simulink model "model"  (R2016b)
settings: Solver=VariableStepAuto  StartTime=0.0  StopTime=par.t12  FixedStep=0.001  RelTol=1e-6
StartFcn:
  | tic;
StopFcn:
  | toc;
values from neighbouring files (symbols this model uses):
  as = rmfield(as,'data')    [PrepareForModel (2).m]    (also in PrepareForModel.m)
  trj = rmfield(trj,'aerodata')    [ImportFromMatAndExcel.m]
undefined symbols (not defined in the file or in its folder): dm
libraries: aerolibschedule x5, simulink_extras x2
settings Model: Creator=admin  LastModifiedBy=ivan_
settings SolverCC: PositivePriorityOrder=on  AutoInsertRateTranBlk=on
settings DataIOCC: LimitDataPoints=on  SaveFormat=Array
settings OptimizationCC: LifeSpan=inf
settings DebuggingCC: SFUnexpectedBacktrackingDiag=warning  SFNoUnconditionalDefaultTransitionDiag=warning  SFExecutionAtInitializationDiag=none
settings HardwareCC: ProdBitPerPointer=32  ProdBitPerSizeT=32  ProdBitPerPtrDiffT=32  ProdLargestAtomicFloat=None  ProdIntDivRoundTo=Undefined  ProdEndianess=Unspecified  ProdWordSize=32  ProdHWDeviceType=32-bit Generic
settings ModelReferenceCC: PropagateSignalLabelsOutOfModel=off
settings GRTTargetCC: TargetLangStandard=C89/C90 (ANSI)  GeneratePreprocessorConditionals=Disable all
settings ConfigComp: CovMetricSettings=dw  CovHtmlReporting=on  CovSaveCumulativeToWorkspaceVar=on  CovSaveSingleToWorkspaceVar=on  CovExternalEMLEnable=off  CovSFcnEnable=off

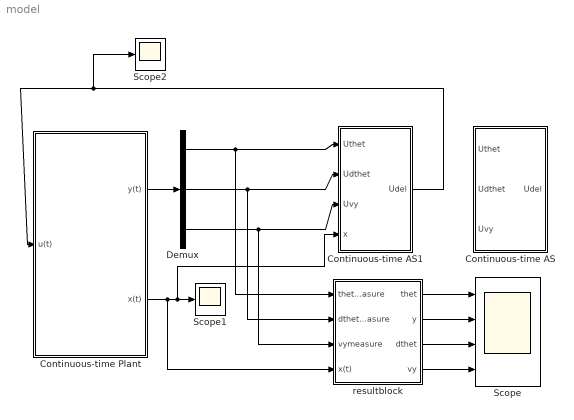
== system model ==
  Continuous-time Plant : Subsystem  VariantControl=Variant
  Continuous-time AS : Subsystem  VariantControl=Variant1
  Continuous-time AS1 : Subsystem  VariantControl=Variant1
  Demux : Demux  Outputs=3
  Scope : Scope  NumInputPorts=4
  Scope1 : Scope
  Scope2 : Scope
  resultblock : Subsystem
  wires:
  Demux/1 -> Continuous-time AS1/1(Uthet), resultblock/1(thetmeasure)
  Demux/2 -> Continuous-time AS1/2(Udthet), resultblock/2(dthetmeasure)
  Demux/3 -> Continuous-time AS1/3(Uvy), resultblock/3(vymeasure)
  Continuous-time Plant/1(y(t)) -> Demux/1
  resultblock/1(thet) -> Scope/1
  resultblock/2(y) -> Scope/2
  resultblock/3(dthet) -> Scope/3
  resultblock/4(vy) -> Scope/4
  Continuous-time Plant/2(x(t)) -> Continuous-time AS1/4("x "), Scope1/1, resultblock/4(x(t))
  Continuous-time AS1/1(Udel) -> Scope2/1, Continuous-time Plant/1(u(t))

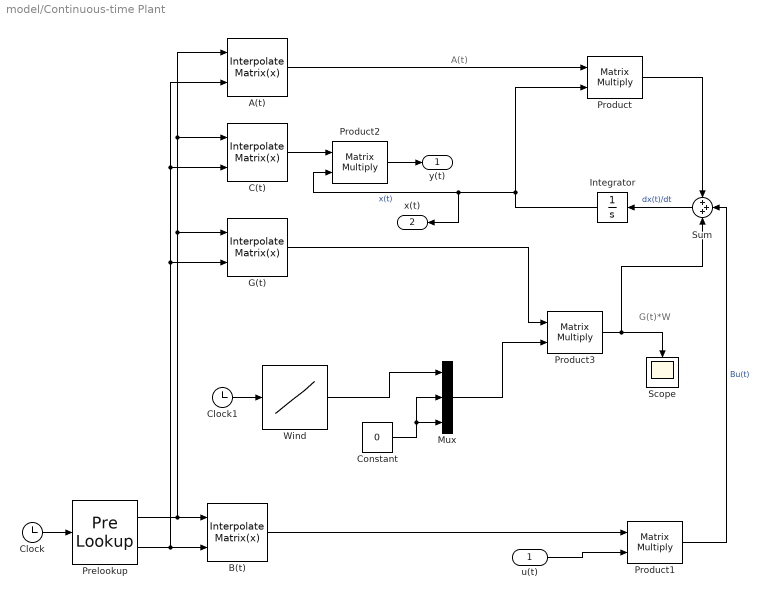
== system model/Continuous-time Plant ==
  note: G(t)*W
  note: A(t)
  u(t) : Inport
  "A(t) " : aerolibschedule/Interpolate Matrix(x)   matrix=dm.A
  B(t) : aerolibschedule/Interpolate Matrix(x)   matrix=dm.B
  C(t) : aerolibschedule/Interpolate Matrix(x)   matrix=dm.C
  Clock : Clock
  Clock1 : Clock
  Constant : Constant  Value=0
  G(t) : aerolibschedule/Interpolate Matrix(x)   matrix=dm.G
  Integrator : Integrator
  Mux : Mux  Inputs=3
  Prelookup : PreLookup  BreakpointsData=dm.t
  Product{,1..3} (4 alike) : Product  Multiplication=Matrix(*)
  Scope : Scope
  Sum : Sum  Inputs=+++
  Wind : Lookup_n-D  NumberOfTableDimensions=1  BreakpointsForDimension1=dm.t  Table=trj.wind  ExtrapMethod=Clip  UseLastTableValue=on  InternalRulePriority=Speed  RndMeth=Simplest  InputSameDT=on
  y(t) : Outport
  x(t) : Outport  Port=2
  wires:
  Sum/1 -> Integrator/1  "dx(t)/dt"
  u(t)/1 -> Product1/2
  Integrator/1 -> Product2/2, x(t)/1, Product/2  "x(t)"
  Product2/1 -> y(t)/1
  Mux/1 -> Product3/2
  Product3/1 -> Sum/3, Scope/1
  G(t)/1 -> Product3/1
  "A(t) "/1 -> Product/1
  B(t)/1 -> Product1/1
  C(t)/1 -> Product2/1
  Wind/1 -> Mux/1
  Prelookup/2 -> "A(t) "/2, C(t)/2, G(t)/2, B(t)/2
  Prelookup/1 -> "A(t) "/1, C(t)/1, G(t)/1, B(t)/1
  Clock/1 -> Prelookup/1
  Product/1 -> Sum/1
  Clock1/1 -> Wind/1
  Product1/1 -> Sum/2  "Bu(t)"
  Constant/1 -> Mux/3, Mux/2

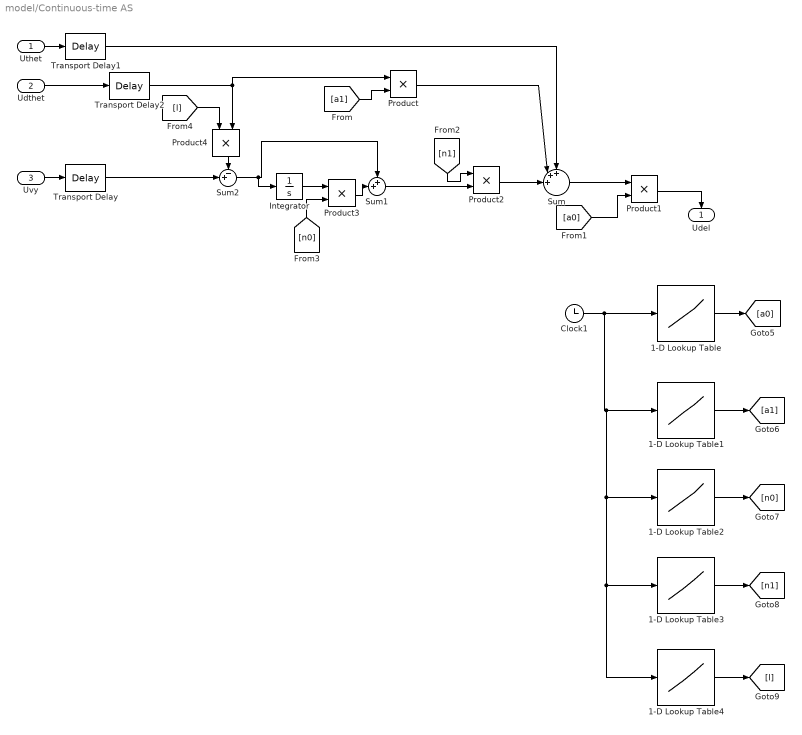
== system model/Continuous-time AS ==
  Uthet : Inport
  Udthet : Inport  Port=2
  Uvy : Inport  Port=3
  1-D Lookup Table : Lookup_n-D  NumberOfTableDimensions=1  BreakpointsForDimension1=as.t  Table=as.a0  ExtrapMethod=Clip  UseLastTableValue=on  InternalRulePriority=Speed  RndMeth=Simplest  InputSameDT=on
  1-D Lookup Table1 : Lookup_n-D  NumberOfTableDimensions=1  BreakpointsForDimension1=as.t  Table=as.a1  ExtrapMethod=Clip  UseLastTableValue=on  InternalRulePriority=Speed  RndMeth=Simplest  InputSameDT=on
  1-D Lookup Table2 : Lookup_n-D  NumberOfTableDimensions=1  BreakpointsForDimension1=as.t  Table=as.n0  ExtrapMethod=Clip  UseLastTableValue=on  InternalRulePriority=Speed  RndMeth=Simplest  InputSameDT=on
  1-D Lookup Table3 : Lookup_n-D  NumberOfTableDimensions=1  BreakpointsForDimension1=as.t  Table=as.n1  ExtrapMethod=Clip  UseLastTableValue=on  InternalRulePriority=Speed  RndMeth=Simplest  InputSameDT=on
  1-D Lookup Table4 : Lookup_n-D  NumberOfTableDimensions=1  BreakpointsForDimension1=as.t  Table=as.l  ExtrapMethod=Clip  UseLastTableValue=on  InternalRulePriority=Speed  RndMeth=Simplest  InputSameDT=on
  Clock1 : Clock
  Integrator : Integrator
  Product{,1..4} (5 alike) : Product
  Sum : Sum  Inputs=+++||
  Sum1 : Sum  Inputs=++|
  Sum2 : Sum  Inputs=-+|
  Transport Delay : TransportDelay  DelayTime=[0.0214]
  Transport Delay1 : TransportDelay  DelayTime=[0.0214]
  Transport Delay2 : TransportDelay  DelayTime=[0.0114]
  Udel : Outport
  wires:
  Sum2/1 -> Integrator/1, Sum1/1
  Sum1/1 -> Product2/2
  Udthet/1 -> Transport Delay2/1
  Sum/1 -> Product1/1
  Product4/1 -> Sum2/1
  Product/1 -> Sum/2
  Uvy/1 -> Transport Delay/1
  Uthet/1 -> Transport Delay1/1
  [a1] -> Product/2
  [a0] -> Product1/2
  Product2/1 -> Sum/3
  Product1/1 -> Udel/1
  [l] -> Product4/1
  [n1] -> Product2/1
  1-D Lookup Table/1 -> [a0]
  1-D Lookup Table1/1 -> [a1]
  1-D Lookup Table2/1 -> [n0]
  1-D Lookup Table3/1 -> [n1]
  1-D Lookup Table4/1 -> [l]
  Clock1/1 -> 1-D Lookup Table4/1, 1-D Lookup Table3/1, 1-D Lookup Table2/1, 1-D Lookup Table1/1, 1-D Lookup Table/1
  [n0] -> Product3/2
  Integrator/1 -> Product3/1
  Product3/1 -> Sum1/2
  Transport Delay/1 -> Sum2/2
  Transport Delay1/1 -> Sum/1
  Transport Delay2/1 -> Product4/2, Product/1

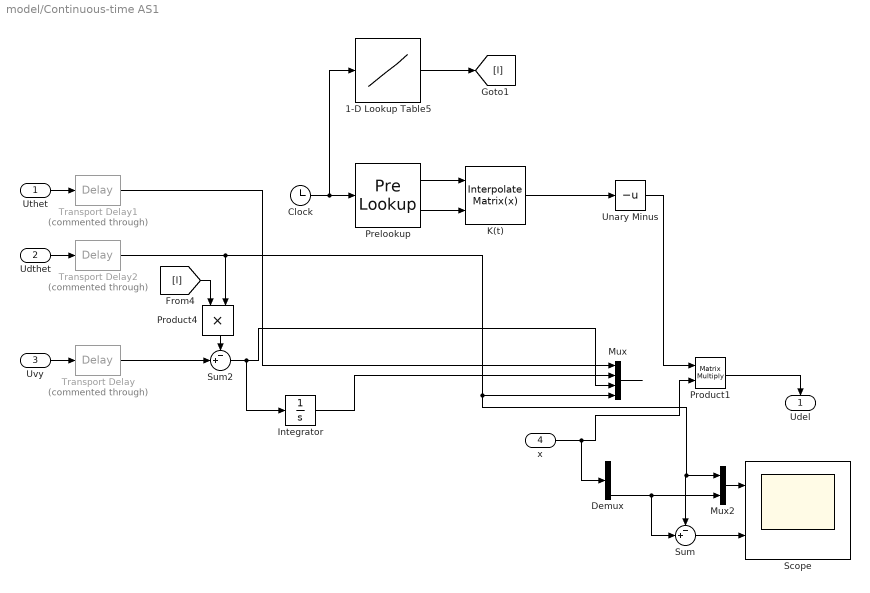
== system model/Continuous-time AS1 ==
  Uthet : Inport
  Udthet : Inport  Port=2
  Uvy : Inport  Port=3
  "x " : Inport  Port=4
  1-D Lookup Table5 : Lookup_n-D  NumberOfTableDimensions=1  BreakpointsForDimension1=as.t  Table=as.l  ExtrapMethod=Clip  UseLastTableValue=on  InternalRulePriority=Speed  RndMeth=Simplest  InputSameDT=on
  Clock : Clock
  Demux : Demux
  Integrator : Integrator
  K(t) : aerolibschedule/Interpolate Matrix(x)   matrix=as.k
  Mux : Mux
  Mux2 : Mux  Inputs=2
  Prelookup : PreLookup  BreakpointsData=dm.t
  Product1 : Product  Multiplication=Matrix(*)
  Product4 : Product
  Scope : Scope  NumInputPorts=2
  Sum : Sum  Inputs=-+|
  Sum2 : Sum  Inputs=-+|
  Transport Delay : TransportDelay  Commented=through  DelayTime=[0.0214]
  Transport Delay1 : TransportDelay  Commented=through  DelayTime=[0.0214]
  Transport Delay2 : TransportDelay  Commented=through  DelayTime=[0.0114]
  Unary Minus : UnaryMinus
  Udel : Outport
  wires:
  Udthet/1 -> Transport Delay2/1
  Product4/1 -> Sum2/1
  Uvy/1 -> Transport Delay/1
  Uthet/1 -> Transport Delay1/1
  K(t)/1 -> Unary Minus/1
  Product1/1 -> Udel/1
  [l] -> Product4/1
  Transport Delay/1 -> Sum2/2
  Transport Delay2/1 -> Product4/2, Sum/1, Mux2/1, Mux/4
  Prelookup/2 -> K(t)/2
  Prelookup/1 -> K(t)/1
  Clock/1 -> 1-D Lookup Table5/1, Prelookup/1
  1-D Lookup Table5/1 -> [l]
  Transport Delay1/1 -> Mux/1
  Integrator/1 -> Mux/2
  Mux/1 -> ?
  Unary Minus/1 -> Product1/1
  "x "/1 -> Demux/1, Product1/2
  Sum2/1 -> Integrator/1, Mux/3
  Demux/4 -> Mux2/2, Sum/2
  Mux2/1 -> Scope/1
  Sum/1 -> Scope/2

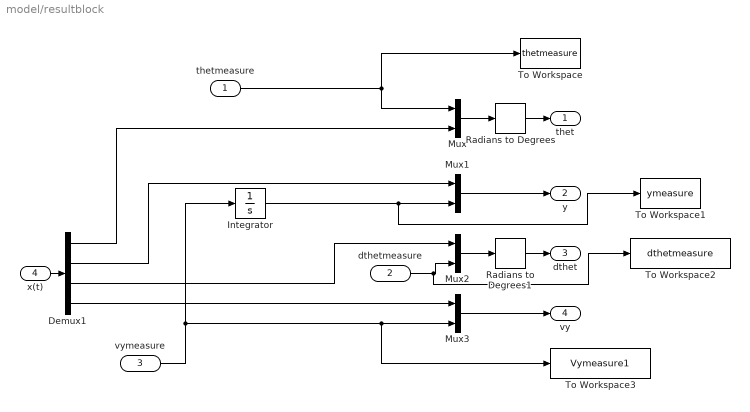
== system model/resultblock ==
  thetmeasure : Inport
  dthetmeasure : Inport  Port=2
  vymeasure : Inport  Port=3
  x(t) : Inport  Port=4
  Demux1 : Demux
  Integrator : Integrator
  Mux{,1..3} (4 alike) : Mux  Inputs=2
  Radians to Degrees : simulink_extras/Transformations/Radians to Degrees
  Radians to Degrees1 : simulink_extras/Transformations/Radians to Degrees
  To Workspace : ToWorkspace  VariableName=thetmeasure  SaveFormat=Structure With Time  SampleTime=-1
  To Workspace1 : ToWorkspace  VariableName=ymeasure  SaveFormat=Structure With Time  SampleTime=-1
  To Workspace2 : ToWorkspace  VariableName=dthetmeasure  SaveFormat=Structure With Time  SampleTime=-1
  To Workspace3 : ToWorkspace  VariableName=Vymeasure1  SaveFormat=Structure With Time  SampleTime=-1
  thet : Outport
  y : Outport  Port=2
  dthet : Outport  Port=3
  vy : Outport  Port=4
  wires:
  x(t)/1 -> Demux1/1
  thetmeasure/1 -> Mux/1, To Workspace/1
  Integrator/1 -> To Workspace1/1, Mux1/2
  dthetmeasure/1 -> To Workspace2/1, Mux2/2
  Demux1/2 -> Mux1/1
  Demux1/3 -> Mux2/1
  Mux/1 -> Radians to Degrees/1
  Demux1/1 -> Mux/2
  Mux3/1 -> vy/1
  Demux1/4 -> Mux3/1
  vymeasure/1 -> Integrator/1, To Workspace3/1, Mux3/2
  Mux1/1 -> y/1
  Mux2/1 -> Radians to Degrees1/1
  Radians to Degrees1/1 -> dthet/1
  Radians to Degrees/1 -> thet/1
